simulink model "auv_model"  (R2021a)
settings: Solver=FixedStepAuto  StartTime=0.0  StopTime=inf  FixedStep=1/100  RelTol=1e-3
undefined symbols (not defined in the file): mpc, physics, simulation
libraries: robotlib x6, simulink x1
settings Model: EnablePacing=on  Creator=lamarre  LastModifiedBy=lamarre
settings SolverCC: AlgebraicLoopSolver=TrustRegion
settings DebuggingCC: SFMachineParentedDataDiag=warning

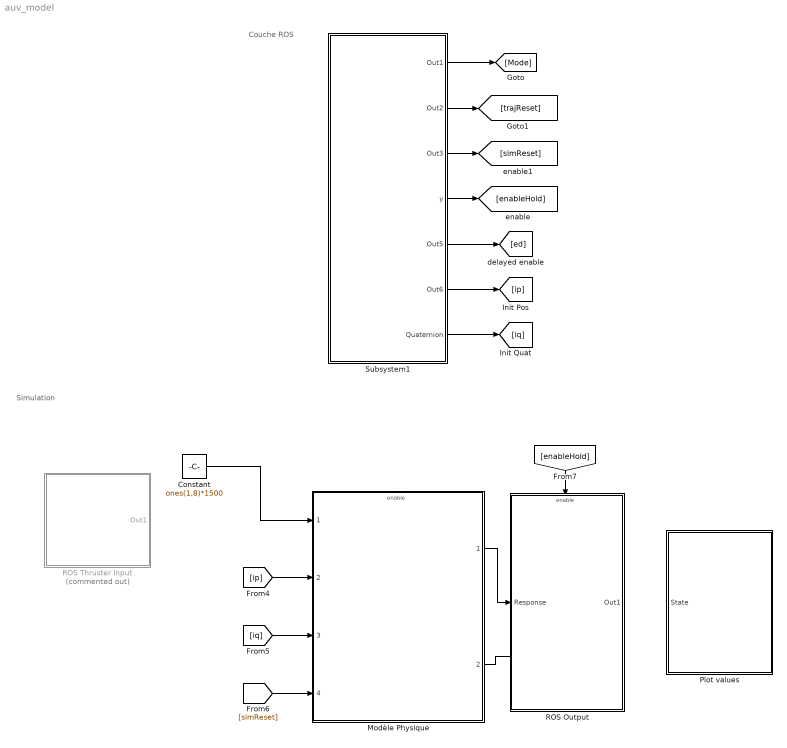
== system auv_model ==
  note: Simulation
  note: Couche ROS
  Constant : Constant  Value=ones(1,8)*1500
  Modèle Physique : Subsystem  InitFcn=|  ReferencedSubsystem=AUVPlant
      | InitController;
      | InitAUVPlant;
  Plot values : Subsystem
  ROS Output : Subsystem
  ROS Thruster Input : Subsystem  Commented=on
  Subsystem1 : Subsystem
  wires:
  [enableHold] -> ROS Output/Enable
  [simReset] -> Modèle Physique/4
  [ip] -> Modèle Physique/2
  [iq] -> Modèle Physique/3
  Modèle Physique/1 -> ROS Output/1(Response)
  ? -> Plot values/1(State)
  Subsystem1/5(Out5) -> [ed]
  Subsystem1/3(Out3) -> [simReset]
  Subsystem1/4(y) -> [enableHold]
  Subsystem1/2(Out2) -> [trajReset]
  Subsystem1/7(Quaternion) -> [iq]
  Subsystem1/1(Out1) -> [Mode]
  Subsystem1/6(Out6) -> [ip]
  Modèle Physique/2 -> ?
  Constant/1 -> Modèle Physique/1

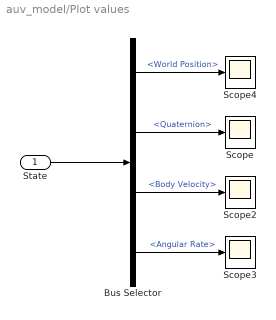
== system auv_model/Plot values ==
  State : Inport
  Bus Selector : BusSelector  OutputSignals=World Position,Quaternion,Body Velocity,Angular Rate
  Scope{,2..4} (4 alike) : Scope
  wires:
  Bus Selector/4 -> Scope3/1  "<Angular Rate>"
  State/1 -> Bus Selector/1
  Bus Selector/2 -> Scope/1  "<Quaternion>"
  Bus Selector/3 -> Scope2/1  "<Body Velocity>"
  Bus Selector/1 -> Scope4/1  "<World Position>"

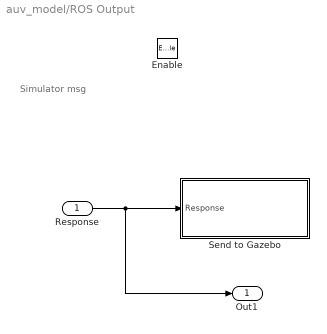
== system auv_model/ROS Output ==
  note: Simulator msg
  Response : Inport
  Enable : EnablePort
  Send to Gazebo : Subsystem  InitFcn=""
  Out1 : Outport
  wires:
  Response/1 -> Out1/1, Send to Gazebo/1(Response)

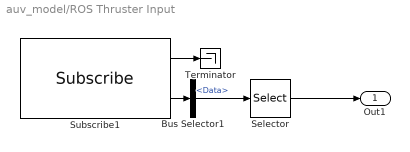
== system auv_model/ROS Thruster Input ==
  Bus Selector1 : BusSelector  OutputSignals=Data
  Selector : Selector  InputPortWidth=128  IndexOptions=Index vector (dialog)  Indices=[1:8]  OutputSizes=1
  Subscribe1 : robotlib/Subscribe  topicSource=Specify your own  topic=/provider_thruster/thruster_pwm  messageType=std_msgs/UInt16MultiArray  SampleTime=-1  legacyBusStruct=off  messageQueueLength=1
  Terminator : Terminator
  Out1 : Outport
  wires:
  Subscribe1/2 -> Bus Selector1/1
  Subscribe1/1 -> Terminator/1
  Bus Selector1/1 -> Selector/1  "<Data>"
  Selector/1 -> Out1/1

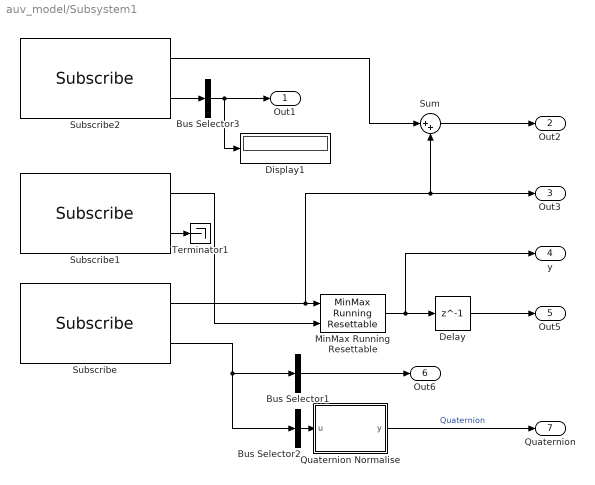
== system auv_model/Subsystem1 ==
  Bus Selector1 : BusSelector  OutputSignals=Position.X,Position.Y,Position.Z  OutputAsBus=on
  Bus Selector2 : BusSelector  OutputSignals=Orientation.W,Orientation.Z,Orientation.Y,Orientation.X  OutputAsBus=on
  Bus Selector3 : BusSelector  OutputSignals=Data  OutputAsBus=on
  Delay : Delay  DelayLength=1
  Display1 : Display
  MinMax Running Resettable : simulink/Math Operations/MinMax Running Resettable  Function=max  vinit=0.0
  Quaternion Normalise : MATLAB Function  TreatAsAtomicUnit=on
  Subscribe : robotlib/Subscribe  topicSource=Select from ROS network  topic=/initial_condition  messageType=geometry_msgs/Pose  SampleTime=mpc.Ts  legacyBusStruct=off  messageQueueLength=1
  Subscribe1 : robotlib/Subscribe  topicSource=Specify your own  topic=/proc_control/kill  messageType=std_msgs/Bool  SampleTime=mpc.Ts  legacyBusStruct=off  messageQueueLength=1
  Subscribe2 : robotlib/Subscribe  topicSource=Specify your own  topic=/proc_control/set_mode  messageType=std_msgs/UInt8  SampleTime=mpc.Ts  legacyBusStruct=off  messageQueueLength=1
  Sum : Sum  Inputs=|++
  Terminator1 : Terminator
  Out1 : Outport
  Out2 : Outport  Port=2
  Out3 : Outport  Port=3
  y : Outport  Port=4
  Out5 : Outport  Port=5
  Out6 : Outport  Port=6
  Quaternion : Outport  Port=7
  wires:
  Bus Selector2/1 -> Quaternion Normalise/1(u)
  Sum/1 -> Out2/1
  Bus Selector3/1 -> Display1/1, Out1/1
  Quaternion Normalise/1(y) -> Quaternion/1  "Quaternion"
  Subscribe/1 -> Out3/1, Sum/2, MinMax Running Resettable/1
  Subscribe1/1 -> MinMax Running Resettable/2
  Subscribe1/2 -> Terminator1/1
  Bus Selector1/1 -> Out6/1
  Subscribe2/2 -> Bus Selector3/1
  Delay/1 -> Out5/1
  Subscribe/2 -> Bus Selector2/1, Bus Selector1/1
  MinMax Running Resettable/1 -> y/1, Delay/1
  Subscribe2/1 -> Sum/1

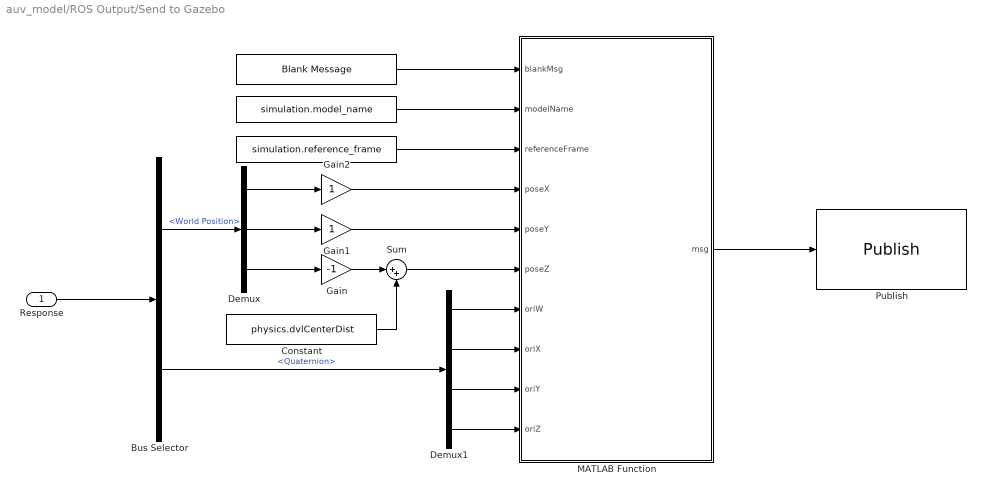
== system auv_model/ROS Output/Send to Gazebo ==
  Response : Inport
  " " : Constant  Value=simulation.model_name  VectorParams1D=off
  "  " : Constant  Value=simulation.reference_frame
  "   " : robotlib/Blank Message  messageClass=Message  entityType=gazebo_msgs/ModelState  messageType=gazebo_msgs/ModelState  SampleTime=1/60  legacyBusStruct=off
  Bus Selector : BusSelector  OutputSignals=World Position,Quaternion
  Constant : Constant  Value=physics.dvlCenterDist
  Demux : Demux  Outputs=3
  Demux1 : Demux
  Gain : Gain  Gain=-1
  Gain1 : Gain
  Gain2 : Gain
  MATLAB Function : MATLAB Function  TreatAsAtomicUnit=on  SystemSampleTime=1/60
  Publish : robotlib/Publish  topicSource=Select from ROS network  topic=/gazebo/set_model_state  messageType=gazebo_msgs/ModelState  legacyBusStruct=off  messageQueueLength=1
      link override SinkBlock: ROSTopic=/gazebo/set_model_state  ROSMessageType=gazebo_msgs/ModelState  SLBusName=SL_Bus_plant_gazebo_msgs_ModelState  ModelName=plant  BlockId=Pub_plant_206
  Sum : Sum  Inputs=|++
  wires:
  Bus Selector/1 -> Demux/1  "<World Position>"
  Demux/1 -> Gain2/1
  Demux/2 -> Gain1/1
  Demux/3 -> Gain/1
  "   "/1 -> MATLAB Function/1(blankMsg)
  "  "/1 -> MATLAB Function/3(referenceFrame)
  " "/1 -> MATLAB Function/2(modelName)
  Gain1/1 -> MATLAB Function/5(poseY)
  Bus Selector/2 -> Demux1/1  "<Quaternion>"
  Demux1/1 -> MATLAB Function/7(oriW)
  Demux1/2 -> MATLAB Function/8(oriX)
  Demux1/3 -> MATLAB Function/9(oriY)
  Demux1/4 -> MATLAB Function/10(oriZ)
  Gain2/1 -> MATLAB Function/4(poseX)
  MATLAB Function/1(msg) -> Publish/1
  Response/1 -> Bus Selector/1
  Gain/1 -> Sum/1
  Sum/1 -> MATLAB Function/6(poseZ)
  Constant/1 -> Sum/2

== matlab function auv_model/Subsystem1/Quaternion Normalise ==
  data: u input size=4; y output size=4
function y = Normalize(u)
%Normailse le quaternions pour éviter la distortions crée par l'erreur de
% de l'intégration.
d=norm(u);
n=u/d;
if isnan(n)
    y=[1;0;0;0];
else
    y = n;
end

== matlab function auv_model/ROS Output/Send to Gazebo/MATLAB Function ==
  data: blankMsg input; msg output Bus: SL_Bus_auv_model_gazebo_msgs_ModelState; modelName input; referenceFrame input; poseX input; poseY input; poseZ input; oriW input; oriX input; oriY input; oriZ input
function msg = assignGazeboModelStateInput(blankMsg, modelName, referenceFrame, poseX, poseY, poseZ, oriW, oriX, oriY, oriZ)
% assignStringInput - Assign a string in a ROS message to specified input string
%
% MSG = assignStringInput(blankMsg, STR) assigns the input string, STR, to
%  a string field in the ROS message, blankMsg, and outputs the updated
%  ROS message.
%
%  Inputs
%    blankMsg: A bus for a 'std_msgs/String' message. This is 
%        used to initialize the output.
%    str: An array of uint8 that will be assigned to the 'Data' field
%        in blankMsg. The entire array is assumed to be a valid sequence of
%        character ASCII values.
% 
%  Outputs:
%    msg: A bus for a 'std_msgs/String' message, with the 'Data'
%        field set to a string.

%   Copyright 2015 The MathWorks, Inc.
%#codegen

% Note: The datatype of 'msg' has been explicitly set to the appropriate 
% Simulink bus type ("Bus: SL_Bus_robotROSMessageUsageExample_std_msgs_String"). 
%
% If the model name is changed, the datatype needs to be changed as well:
%   1) Click "Edit Data" in the Editor toolstrip to open "Ports and Data Manager"
%   2) Select "msg". From the "Type" dropdown, select "--- Refresh data types ---"
%   3) Set datatype to "Bus: SL_Bus_<modelname>_std_msgs_String"
   
msg = blankMsg;

strLength = length(modelName);
msg.ModelName(1:strLength) = modelName;
msg.ModelName_SL_Info.CurrentLength = uint32(strLength);

strLength = length(referenceFrame);
msg.ReferenceFrame(1:strLength) = referenceFrame;
msg.ReferenceFrame_SL_Info.CurrentLength = uint32(strLength);

msg.Pose.Position.X = poseX;
msg.Pose.Position.Y = poseY;
msg.Pose.Position.Z = poseZ;

msg.Pose.Orientation.X = oriX;
msg.Pose.Orientation.Y = oriY;
msg.Pose.Orientation.Z = oriZ;
msg.Pose.Orientation.W = oriW;
